simulink model "ids_sim"  (R2023b)
settings: Solver=VariableStepAuto  StartTime=0.0  StopTime=inf  RelTol=1e-3
undefined symbols (not defined in the file or in its folder): canChannel, sawtooth, square
libraries: canlib x7, canmsglib x6, simulink x3
settings Model: LastModifiedBy=huyang

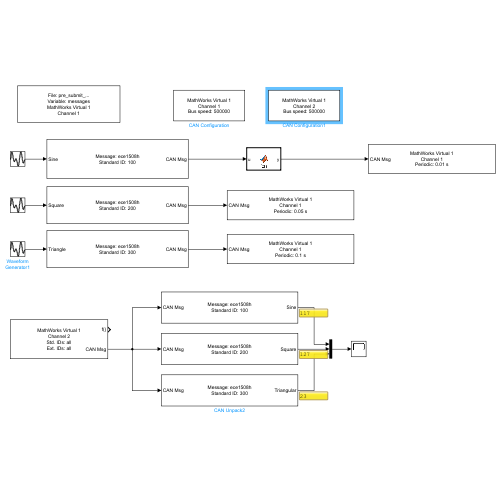
[thumbnail: Simulink's stored preview of the top-level diagram]
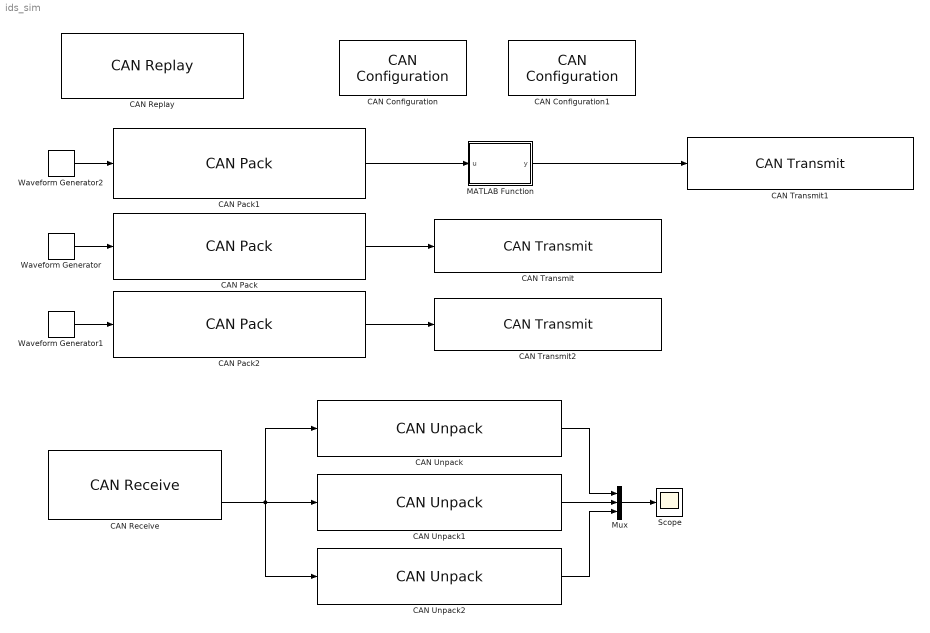
== system ids_sim ==
  CAN Configuration : canlib/CAN Configuration  BlockHandle=5492.0002  Device=MathWorks Virtual 1 (Channel 1)  DeviceMenu=MathWorks Virtual 1 (Channel 1)  ObjConstructor=canChannel('MathWorks', 'Virtual 1', 1)  BusSpeed=500000  EnableBitParameters=off  AckMode=Normal
  CAN Configuration1 : canlib/CAN Configuration  BlockHandle=5492.0002  Device=MathWorks Virtual 1 (Channel 2)  DeviceMenu=MathWorks Virtual 1 (Channel 2)  ObjConstructor=canChannel('MathWorks', 'Virtual 1', 2)  BusSpeed=500000  EnableBitParameters=off  AckMode=Normal
  CAN Pack : canmsglib/CAN Pack  MsgList=(none)  MsgName=ece1508h  MsgIDType=Standard (11-bit identifier)  MsgIdentifier=200  MsgLength=8  Remote=off  ApplyMinMax=off  BusOutput=off  SignalInfo={ 'Square', '8', '8', 'LE', 'signed', 'Standard', '0', '1', '0', '-Inf', 'Inf' }
      settings: LibrarySourceBlock=canlib/CAN Pack  DataFormat=manually specified signals
  CAN Pack1 : canmsglib/CAN Pack  MsgList=(none)  MsgName=ece1508h  MsgIDType=Standard (11-bit identifier)  MsgIdentifier=100  MsgLength=8  Remote=off  ApplyMinMax=off  BusOutput=off  SignalInfo={ 'Sine', '0', '8', 'LE', 'signed', 'Standard', '0', '1', '0', '-Inf', 'Inf' }
      settings: LibrarySourceBlock=canlib/CAN Pack  DataFormat=manually specified signals
  CAN Pack2 : canmsglib/CAN Pack  MsgList=(none)  MsgName=ece1508h  MsgIDType=Standard (11-bit identifier)  MsgIdentifier=300  MsgLength=8  Remote=off  ApplyMinMax=off  BusOutput=off  SignalInfo={ 'Triangle', '16', '8', 'LE', 'signed', 'Standard', '0', '1', '0', '-Inf', 'Inf' }
      settings: LibrarySourceBlock=canlib/CAN Pack  DataFormat=manually specified signals
  CAN Receive : canlib/CAN Receive  BlockHandle=5494.0002  Device=MathWorks Virtual 1 (Channel 2)  DeviceMenu=MathWorks Virtual 1 (Channel 2)  ObjConstructor=canChannel('MathWorks', 'Virtual 1', 2)  EnableStandardIDsFilter=off  StdIDsCombo=Allow all  StandardIDs=100  EnableExtendedIDsFilter=off  ExtIDsCombo=Allow all  ExtendedIDs=0  SampleTime=0.00001  MsgsPerTimestep=all  InternalFilterUpdateStatus=on  BusOutput=off
  CAN Replay : canlib/CAN Replay  BlockHandle=5425.0002  FullPathFileName=Z:\Desktop\Courses\ECE1508-Cybersecurity\final project\code\pre_submit_d.mat  FileName=pre_submit_d.mat  VariableName=messages  NoTimesReplay=Inf  ReplayTo=CAN Bus  DeviceMenu=MathWorks Virtual 1 (Channel 1)  Device=MathWorks Virtual 1 (Channel 1)  ObjConstructor=canChannel('MathWorks', 'Virtual 1', 1)  SampleTime=0.01  BusOutput=off
  CAN Transmit : canlib/CAN Transmit  BlockHandle=5495.0002  Device=MathWorks Virtual 1 (Channel 1)  DeviceMenu=MathWorks Virtual 1 (Channel 1)  ObjConstructor=canChannel('MathWorks', 'Virtual 1', 1)  EnableEventTransmit=off  EnablePeriodicTransmit=on  MessagePeriod=0.05
  CAN Transmit1 : canlib/CAN Transmit  BlockHandle=5495.0002  Device=MathWorks Virtual 1 (Channel 1)  DeviceMenu=MathWorks Virtual 1 (Channel 1)  ObjConstructor=canChannel('MathWorks', 'Virtual 1', 1)  EnableEventTransmit=off  EnablePeriodicTransmit=on  MessagePeriod=0.010
  CAN Transmit2 : canlib/CAN Transmit  BlockHandle=5495.0002  Device=MathWorks Virtual 1 (Channel 1)  DeviceMenu=MathWorks Virtual 1 (Channel 1)  ObjConstructor=canChannel('MathWorks', 'Virtual 1', 1)  EnableEventTransmit=off  EnablePeriodicTransmit=on  MessagePeriod=0.1
  CAN Unpack : canmsglib/CAN Unpack  MsgList=(none)  MsgName=ece1508h  MsgIDType=Standard (11-bit identifier)  MsgIdentifier=100  MsgLength=8  SignalInfo={ 'Sine', '0', '8', 'LE', 'signed', 'Standard', '0', '1', '0', '-Inf', 'Inf' }  IDPort=off  TimestampPort=off  ErrorPort=off  RemotePort=off  LengthPort=off  StatusPort=off  ApplyMinMax=off
      settings: LibrarySourceBlock=canlib/CAN Unpack
  CAN Unpack1 : canmsglib/CAN Unpack  MsgList=(none)  MsgName=ece1508h  MsgIDType=Standard (11-bit identifier)  MsgIdentifier=200  MsgLength=8  SignalInfo={ 'Square', '8', '8', 'LE', 'signed', 'Standard', '0', '1', '0', '-Inf', 'Inf' }  IDPort=off  TimestampPort=off  ErrorPort=off  RemotePort=off  LengthPort=off  StatusPort=off  ApplyMinMax=off
      settings: LibrarySourceBlock=canlib/CAN Unpack
  CAN Unpack2 : canmsglib/CAN Unpack  MsgList=(none)  MsgName=ece1508h  MsgIDType=Standard (11-bit identifier)  MsgIdentifier=300  MsgLength=8  SignalInfo={ 'Triangular', '16', '8', 'LE', 'signed', 'Standard', '0', '1', '0', '-Inf', 'Inf' }  IDPort=off  TimestampPort=off  ErrorPort=off  RemotePort=off  LengthPort=off  StatusPort=off  ApplyMinMax=off
      settings: LibrarySourceBlock=canlib/CAN Unpack
  MATLAB Function : MATLAB Function  TreatAsAtomicUnit=on
  Mux : Mux  Inputs=3
  Scope : Scope
  Waveform Generator : simulink/Sources/Waveform Generator  OutMin=[]  OutMax=[]  OutDataTypeStr=double  SelectedSignal=1  Signals=square('Amplitude', 128, 'Frequency', 20)  BlockNames=MultiportSwitch_2a05d9e74a11433  SampleTime=0.001
  Waveform Generator1 : simulink/Sources/Waveform Generator  OutMin=[]  OutMax=[]  OutDataTypeStr=double  SelectedSignal=1  Signals=sawtooth('Amplitude', 128, 'Frequency', 20)  BlockNames=MultiportSwitch_033f49ba66a5494  SampleTime=0.001
  Waveform Generator2 : simulink/Sources/Waveform Generator  OutMin=[]  OutMax=[]  OutDataTypeStr=double  SelectedSignal=1  Signals=sin('Amplitude', 128, 'Frequency', 20)  BlockNames=MultiportSwitch_801753d8cef1454  SampleTime=0.001
  wires:
  CAN Pack/1 -> CAN Transmit/1
  CAN Receive/2 -> CAN Unpack/1, CAN Unpack1/1, CAN Unpack2/1
  Mux/1 -> Scope/1
  CAN Unpack/1 -> Mux/1
  Waveform Generator/1 -> CAN Pack/1
  CAN Unpack1/1 -> Mux/2
  CAN Unpack2/1 -> Mux/3
  Waveform Generator2/1 -> CAN Pack1/1
  Waveform Generator1/1 -> CAN Pack2/1
  CAN Pack2/1 -> CAN Transmit2/1
  CAN Pack1/1 -> MATLAB Function/1(u)
  MATLAB Function/1(y) -> CAN Transmit1/1

== matlab function ids_sim/MATLAB Function ==
  data: u input; y output
function y = fcn(u)

y = u;
